simulink model "sat_orbit_no_control_SIM"  (R2019b)
settings: Solver=ode45  StartTime=0.0  StopTime=15000.0  MaxStep=0.009  RelTol=1e-8
settings Model: Creator=Hector  LastModifiedBy=Hector
settings SolverCC: AlgebraicLoopSolver=LineSearch

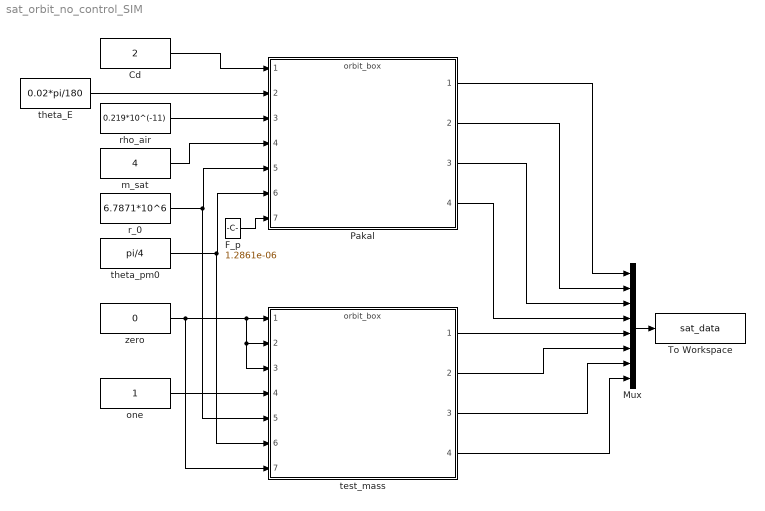
== system sat_orbit_no_control_SIM ==
  Cd : Constant  Value=2
  F_p : Constant  Value=1.2861e-06
  Mux : Mux  Inputs=8
  Pakal : ModelReference  ModelNameDialog=orbit_box.slx  SimulationMode=Normal  ModelReferenceVersion=1.38
  To Workspace : ToWorkspace  VariableName=sat_data  SampleTime=-1
  m_sat : Constant  Value=4
  one : Constant
  r_0 : Constant  Value=6.7871*10^6
  rho_air : Constant  Value=0.219*10^(-11)
  test_mass : ModelReference  ModelNameDialog=orbit_box.slx  SimulationMode=Normal  ModelReferenceVersion=1.38
  theta_E : Constant  Value=0.02*pi/180
  theta_pm0 : Constant  Value=pi/4
  zero : Constant  Value=0
  wires:
  Cd/1 -> Pakal/1
  rho_air/1 -> Pakal/3
  m_sat/1 -> Pakal/4
  r_0/1 -> test_mass/5, Pakal/5
  theta_pm0/1 -> test_mass/6, Pakal/6
  Pakal/2 -> Mux/2
  theta_E/1 -> Pakal/2
  Pakal/1 -> Mux/1
  Mux/1 -> To Workspace/1
  F_p/1 -> Pakal/7
  Pakal/3 -> Mux/3
  Pakal/4 -> Mux/4
  zero/1 -> test_mass/7, test_mass/3, test_mass/2, test_mass/1
  one/1 -> test_mass/4
  test_mass/1 -> Mux/5
  test_mass/2 -> Mux/6
  test_mass/3 -> Mux/7
  test_mass/4 -> Mux/8
